simulink model "fourth"  (Simulink 8.6)
settings: Solver=ode23tb  StartTime=0.0  StopTime=1  MaxStep=1e-4  RelTol=1e-3
libraries: powerlib x7, powerlib_extras x3, aerolibobsolete x1
settings Model: Creator=lenovo  LastModifiedBy=Administrator
settings OptimizationCC: InitFltsAndDblsToZero=on
settings DebuggingCC: SaveWithParameterizedLinksMsg=none  SignalResolutionControl=TryResolveAllWithWarning  MultiTaskDSMMsg=warning  MultiTaskCondExecSysMsg=none  FcnCallInpInsideContextMsg=UseLocalSettings
settings GRTTargetCC: TargetFcnLib=ansi_tfl_tmw.mat

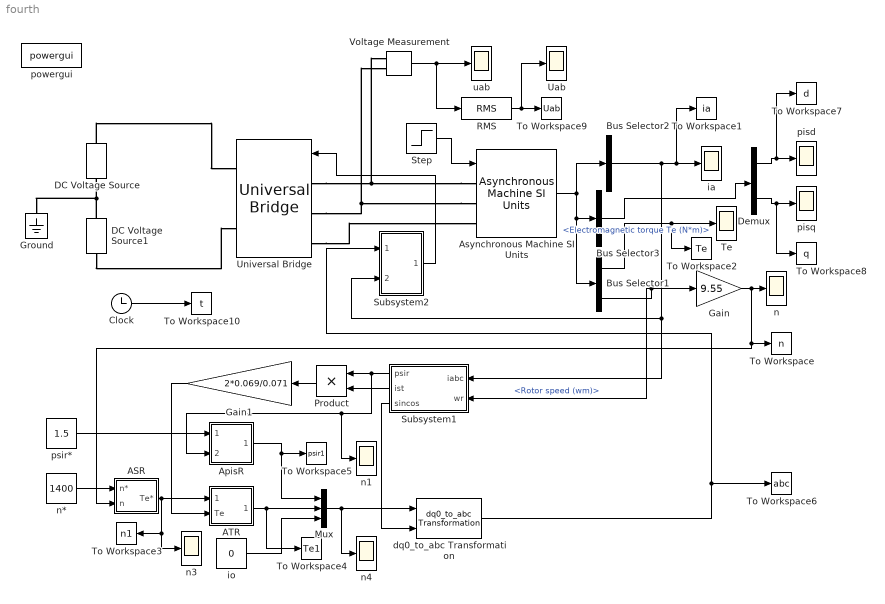
== system fourth ==
  ASR : Subsystem
  ATR : Subsystem
  ApisR : Subsystem
  Asynchronous Machine SI Units : powerlib/Machines/Asynchronous Machine SI Units  RotorType=Squirrel-cage  PresetModel=No  MechanicalLoad=Torque Tm  ShowDetailedParameters=on  ReferenceFrame=Rotor  Units=SI  MeasurementBus=off  NominalParameters=[3730 380 50]  Stator=[0.435 0.002]  Rotor=[0.816 0.002]  Cage1=[0.4155 0.002066]  Cage2=[0.4168 0.0003495]  Lm=0.069  Mechanical=[0.19 0.005752 2]  PolePairs=2  InitialConditions="[ 1,0   0,0,0   0,0,0 ]"  SimulateSaturation=off  Saturation=[9.9249,19.6672,38.0377,51.3988,69.2824,105.1337,152.5532,214.2421,303.1917;230, 322, 414, 460, 506, 552, 598, 644, 690]  LoadFlowParameters=0  TsPowergui=0  TsBlock=-1  IterativeModel=Forward Euler  Pmec=1.492e+006
  Bus Selector1 : BusSelector  OutputSignals=Mechanical.Electromagnetic torque Te (N*m),Mechanical.Rotor speed (wm)
  Bus Selector2 : BusSelector  OutputSignals=Stator measurements.Stator current is_a (A),Stator measurements.Stator current is_b (A),Stator measurements.Stator current is_c (A)  OutputAsBus=on
  Bus Selector3 : BusSelector  OutputSignals=Stator measurements.Stator flux phis_q (V s),Stator measurements.Stator flux phis_d (V s)  OutputAsBus=on
  Clock : Clock
  DC Voltage Source : powerlib/Electrical Sources/DC Voltage Source  Amplitude=205  Measurements=None
  DC Voltage Source1 : powerlib/Electrical Sources/DC Voltage Source  Amplitude=205  Measurements=None
  Demux : Demux  Outputs=2
  Gain : Gain  Gain=9.55
  Gain1 : Gain  Gain=2*0.069/0.071
  Ground : powerlib/Elements/Ground  LConnTagsString=a
  Mux : Mux  Inputs=3
  Product : Product  RndMeth=Zero
  RMS : powerlib_extras/Measurements/RMS  f1=60
  Step : Step  Time=0.6  After=60  SampleTime=0
  Subsystem1 : Subsystem
  Subsystem2 : Subsystem
  Te : Scope
  To Workspace : ToWorkspace  VariableName=n  SampleTime=-1
  To Workspace1 : ToWorkspace  VariableName=ia  SampleTime=-1
  To Workspace10 : ToWorkspace  VariableName=t  SampleTime=-1
  To Workspace2 : ToWorkspace  VariableName=Te  SampleTime=-1
  To Workspace3 : ToWorkspace  VariableName=n1  SampleTime=-1
  To Workspace4 : ToWorkspace  VariableName=Te1  SampleTime=-1
  To Workspace5 : ToWorkspace  VariableName=psir1  SampleTime=-1
  To Workspace6 : ToWorkspace  VariableName=abc  SampleTime=-1
  To Workspace7 : ToWorkspace  VariableName=d  SampleTime=-1
  To Workspace8 : ToWorkspace  VariableName=q  SampleTime=-1
  To Workspace9 : ToWorkspace  VariableName=Uab  SampleTime=-1
  Uab : Scope
  Universal Bridge : powerlib/Power Electronics/Universal Bridge  Arms=3  SnubberResistance=1e5  SnubberCapacitance=inf  Device=IGBT / Diodes  Ron=1e-3  Lon=0  ForwardVoltages="[  0  0  ]"  ForwardVoltage=0  GTOparameters=[ 10e-6 , 20e-6 ]  IGBTparameters=[ 1e-6 , 2e-6 ]  Measurements=None  Measurements_2=None  converterType=Rectifier
  Voltage Measurement : powerlib/Measurements/Voltage Measurement  PhasorSimulation=off  OutputType=Complex  PSBequivalent=0
  dq0_to_abc Transformation : powerlib_extras/Measurements/dq0_to_abc Transformation
  ia : Scope
  io : Constant  Value=0
  n{,1,3..4} (4 alike) : Scope
  n* : Constant  Value=1400
  pisd : Scope
  pisq : Scope
  powergui : powerlib/powergui  SimulationMode=Discrete  SolverType=Tustin/Backward Euler (TBE)  SampleTime=1e-4  frequency=60  SPID=off  DisableSnubberDevices=off  DisableRonSwitches=off  DisableVfSwitches=off  SwTol=0  DisplayEquations=off  Interpol=off  ExternalGateDelay=off  methode=off  Ts=0  FunctionMessages=off  echomessages=off  HookPort=off  EnableUseOfTLC=off  x0status=blocks  frequencyindice=50  Pbase=100e6  ErrMax=1e-4  Iterations=50  UnitsV=kV  UnitsW=MW  buscounter=0  RestoreLinks=warning  ResistiveCurrentMeasurement=off  Frange=[0:2:500]  Ylog=off  Xlog=on  ShowGrid=off  save=off  variable=ZData  ZoomFFT=on  StartTime=0.0  cycles=1  DisplayStyle=1  fundamental=60  FreqAxis=off  MaxFrequency=1000  frequencyindicesteady=1  RmsSteady=1  display=off
  psir* : Constant  Value=1.5
  uab : Scope
  wires:
  n*/1 -> ASR/1(n*)
  ASR/1(Te*) -> ATR/1(Te*), n3/1, To Workspace3/1
  ATR/1(ist*) -> Mux/2, To Workspace4/1
  io/1 -> Mux/3
  ApisR/1(ism*) -> Mux/1, To Workspace5/1
  psir*/1 -> ApisR/1(psir*)
  Mux/1 -> dq0_to_abc Transformation/1, n4/1
  Subsystem1/3(sincos) -> dq0_to_abc Transformation/2
  Subsystem1/2(ist) -> Product/2
  Subsystem1/1(psir) -> ApisR/2(psir), n1/1, Product/1
  Gain1/1 -> ATR/2(Te)
  Asynchronous Machine SI Units/1 -> Bus Selector1/1, Bus Selector3/1, Bus Selector2/1
  Bus Selector1/2 -> Subsystem1/2(wr), Gain/1  "<Rotor speed (wm)>"
  Bus Selector2/1 -> Subsystem1/1(iabc), Subsystem2/2(iabc), ia/1, To Workspace1/1
  Bus Selector1/1 -> Te/1, To Workspace2/1  "<Electromagnetic torque Te (N*m)>"
  Gain/1 -> n/1, ASR/2(n), To Workspace/1
  dq0_to_abc Transformation/1 -> Subsystem2/1(i*abc), To Workspace6/1
  Subsystem2/1(pulses) -> Universal Bridge/1
  Bus Selector3/1 -> Demux/1
  Demux/1 -> pisd/1, To Workspace7/1
  Demux/2 -> pisq/1, To Workspace8/1
  Voltage Measurement/1 -> uab/1, RMS/1
  Step/1 -> Asynchronous Machine SI Units/1
  Product/1 -> Gain1/1
  RMS/1 -> To Workspace9/1, Uab/1
  Clock/1 -> To Workspace10/1
  connections:
  DC Voltage Source1/RConn1 -- DC Voltage Source/LConn1 -- Ground/LConn1
  Asynchronous Machine SI Units/LConn1 -- Universal Bridge/LConn1 -- Voltage Measurement/LConn1
  Asynchronous Machine SI Units/LConn2 -- Universal Bridge/LConn2 -- Voltage Measurement/LConn2
  Universal Bridge/LConn3 -- Asynchronous Machine SI Units/LConn3
  DC Voltage Source/RConn1 -- Universal Bridge/RConn1
  DC Voltage Source1/LConn1 -- Universal Bridge/RConn2

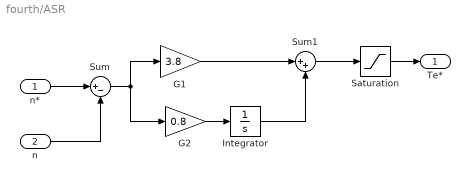
== system fourth/ASR ==
  n* : Inport
  n : Inport  Port=2
  G1 : Gain  Gain=3.8
  G2 : Gain  Gain=0.8
  Integrator : Integrator  LimitOutput=on  UpperSaturationLimit=80  LowerSaturationLimit=-80
  Saturation : Saturate  UpperLimit=75  LowerLimit=-75
  Sum : Sum  Inputs=|+-
  Sum1 : Sum  Inputs=|++
  Te* : Outport
  wires:
  Saturation/1 -> Te*/1
  Sum1/1 -> Saturation/1
  Integrator/1 -> Sum1/2
  G1/1 -> Sum1/1
  G2/1 -> Integrator/1
  n/1 -> Sum/2
  Sum/1 -> G2/1, G1/1
  n*/1 -> Sum/1

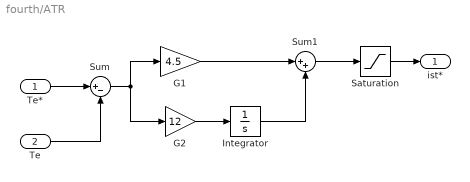
== system fourth/ATR ==
  Te* : Inport
  Te : Inport  Port=2
  G1 : Gain  Gain=4.5
  G2 : Gain  Gain=12
  Integrator : Integrator  LimitOutput=on  UpperSaturationLimit=60  LowerSaturationLimit=-60
  Saturation : Saturate  UpperLimit=60  LowerLimit=-60
  Sum : Sum  Inputs=|+-
  Sum1 : Sum  Inputs=|++
  ist* : Outport
  wires:
  Saturation/1 -> ist*/1
  Sum1/1 -> Saturation/1
  Integrator/1 -> Sum1/2
  G1/1 -> Sum1/1
  G2/1 -> Integrator/1
  Te/1 -> Sum/2
  Sum/1 -> G2/1, G1/1
  Te*/1 -> Sum/1

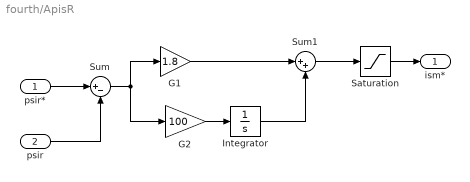
== system fourth/ApisR ==
  psir* : Inport
  psir : Inport  Port=2
  G1 : Gain  Gain=1.8
  G2 : Gain  Gain=100
  Integrator : Integrator  LimitOutput=on  UpperSaturationLimit=15  LowerSaturationLimit=-15
  Saturation : Saturate  UpperLimit=13  LowerLimit=-13
  Sum : Sum  Inputs=|+-
  Sum1 : Sum  Inputs=|++
  ism* : Outport
  wires:
  Saturation/1 -> ism*/1
  Sum1/1 -> Saturation/1
  Integrator/1 -> Sum1/2
  G1/1 -> Sum1/1
  G2/1 -> Integrator/1
  psir/1 -> Sum/2
  Sum/1 -> G2/1, G1/1
  psir*/1 -> Sum/1

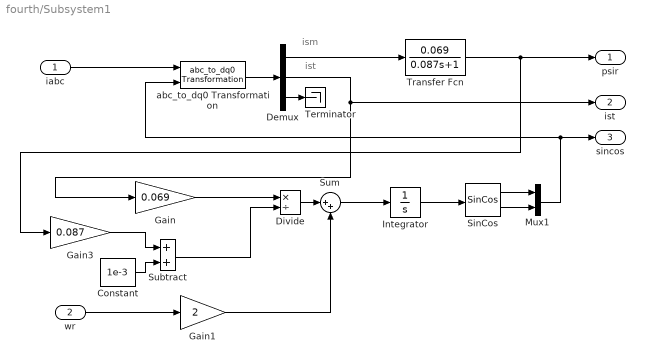
== system fourth/Subsystem1 ==
  note: ist
  note: ism
  iabc : Inport
  wr : Inport  Port=2
  Constant : Constant  Value=1e-3
  Demux : Demux  Outputs=3
  Divide : Product  Inputs=*/
  Gain : Gain  Gain=0.069
  Gain1 : Gain  Gain=2
  Gain3 : Gain  Gain=0.087
  Integrator : Integrator
  Mux1 : Mux  Inputs=2
  SinCos : aerolibobsolete/SinCos
  Subtract : Sum
  Sum : Sum  Inputs=|++
  Terminator : Terminator
  Transfer Fcn : TransferFcn  Numerator=[0.069]  Denominator=[0.087 1]
  abc_to_dq0 Transformation : powerlib_extras/Measurements/abc_to_dq0 Transformation
  psir : Outport
  ist : Outport  Port=2
  sincos : Outport  Port=3
  wires:
  Mux1/1 -> abc_to_dq0 Transformation/2, sincos/1
  SinCos/2 -> Mux1/2
  SinCos/1 -> Mux1/1
  Demux/3 -> Terminator/1
  Demux/2 -> ist/1, Gain/1
  Integrator/1 -> SinCos/1
  Sum/1 -> Integrator/1
  Gain1/1 -> Sum/2
  wr/1 -> Gain1/1
  Transfer Fcn/1 -> psir/1, Gain3/1
  Demux/1 -> Transfer Fcn/1
  abc_to_dq0 Transformation/1 -> Demux/1
  iabc/1 -> abc_to_dq0 Transformation/1
  Gain/1 -> Divide/1
  Subtract/1 -> Divide/2
  Constant/1 -> Subtract/2
  Gain3/1 -> Subtract/1
  Divide/1 -> Sum/1

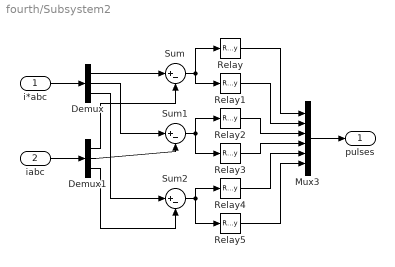
== system fourth/Subsystem2 ==
  i*abc : Inport
  iabc : Inport  Port=2
  Demux : Demux  Outputs=3
  Demux1 : Demux  Outputs=3
  Mux3 : Mux  Inputs=6
  Relay : Relay  OnSwitchValue=0.5  OffSwitchValue=-0.5
  Relay1 : Relay  OnSwitchValue=0.5  OffSwitchValue=-0.5  OnOutputValue=0  OffOutputValue=1
  Relay2 : Relay  OnSwitchValue=0.5  OffSwitchValue=-0.5
  Relay3 : Relay  OnSwitchValue=0.5  OffSwitchValue=-0.5  OnOutputValue=0  OffOutputValue=1
  Relay4 : Relay  OnSwitchValue=0.5  OffSwitchValue=-0.5
  Relay5 : Relay  OnSwitchValue=0.5  OffSwitchValue=-0.5  OnOutputValue=0  OffOutputValue=1
  Sum : Sum  Inputs=|+-
  Sum1 : Sum  Inputs=|+-
  Sum2 : Sum  Inputs=|+-
  pulses : Outport
  wires:
  Mux3/1 -> pulses/1
  Relay5/1 -> Mux3/6
  Relay4/1 -> Mux3/5
  Relay3/1 -> Mux3/4
  Relay2/1 -> Mux3/3
  Relay1/1 -> Mux3/2
  Relay/1 -> Mux3/1
  Sum2/1 -> Relay4/1, Relay5/1
  Sum1/1 -> Relay3/1, Relay2/1
  Sum/1 -> Relay1/1, Relay/1
  Demux1/3 -> Sum2/2
  Demux1/2 -> Sum1/2
  Demux1/1 -> Sum/2
  Demux/3 -> Sum2/1
  Demux/2 -> Sum1/1
  Demux/1 -> Sum/1
  iabc/1 -> Demux1/1
  i*abc/1 -> Demux/1
